simulink model "simple_control"  (R2022b)
settings: Solver=FixedStepDiscrete  StartTime=0.0  StopTime=300  FixedStep=0.01  RelTol=1e-3
model workspace (MAT data in the model file):
  BASE_LENGTH = 0.05
libraries: mobileRoboticsTrainingLib x7
settings Model: NumberOfSteps=10  PacingRate=0.300000  Creator=Amin Fadel  LastModifiedBy=Amin Fadel

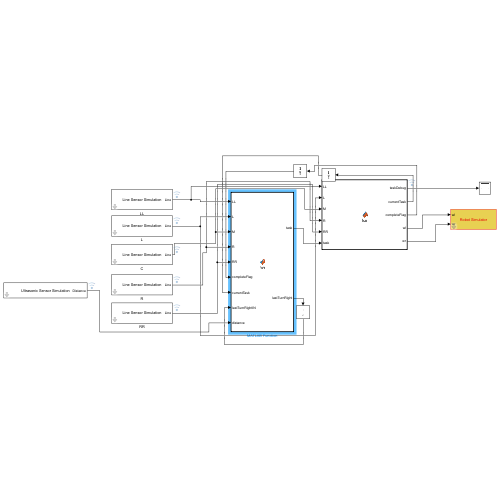
[thumbnail: Simulink's stored preview of the top-level diagram]
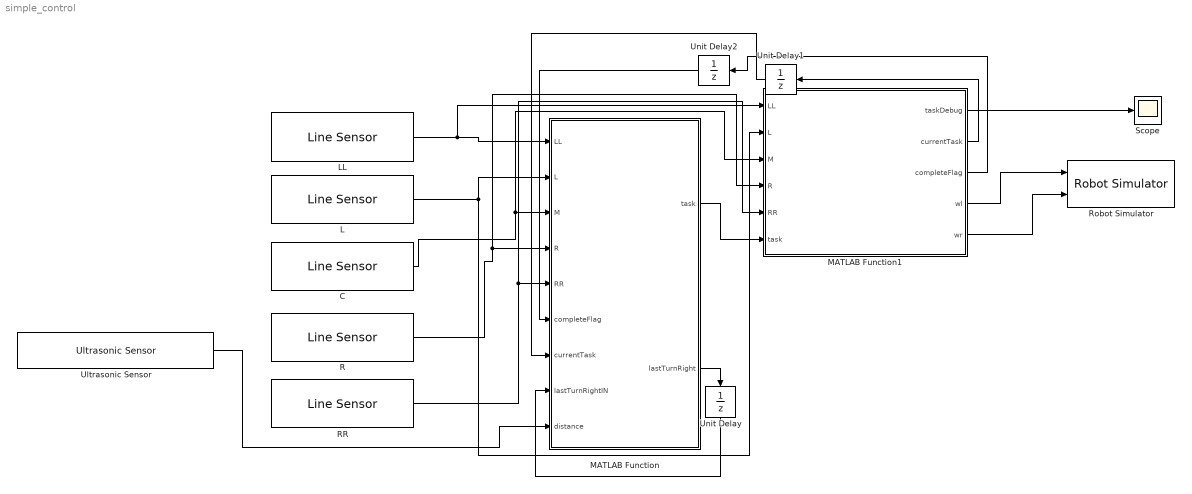
== system simple_control ==
  C : mobileRoboticsTrainingLib/Line Sensor  mapVariable=mapForSim  envVal=0  lineVal=1  sensOff=[BASE_LENGTH+0.05 0]
      settings: SourceProductName=Mobile Robotics Training Library
  L : mobileRoboticsTrainingLib/Line Sensor  mapVariable=mapForSim  envVal=0  lineVal=1  sensOff=[BASE_LENGTH 0.04]
      settings: SourceProductName=Mobile Robotics Training Library
  LL : mobileRoboticsTrainingLib/Line Sensor  mapVariable=mapForSim  envVal=0  lineVal=1  sensOff=[BASE_LENGTH 0.1]
      settings: SourceProductName=Mobile Robotics Training Library
  MATLAB Function : MATLAB Function  TreatAsAtomicUnit=on
  MATLAB Function1 : MATLAB Function  TreatAsAtomicUnit=on
  R : mobileRoboticsTrainingLib/Line Sensor  mapVariable=mapForSim  envVal=0  lineVal=1  sensOff=[BASE_LENGTH -0.04]
      settings: SourceProductName=Mobile Robotics Training Library
  RR : mobileRoboticsTrainingLib/Line Sensor  mapVariable=mapForSim  envVal=0  lineVal=1  sensOff=[BASE_LENGTH -0.1]
      settings: SourceProductName=Mobile Robotics Training Library
  Robot Simulator : mobileRoboticsTrainingLib/Robot Simulator  Priority=99  mapVar=mapForSim  startX=0.10496  startY=1.4665  startTheta=0  axleLength=0.1  wheelR=0.05
  Scope : Scope
  Ultrasonic Sensor : mobileRoboticsTrainingLib/Ultrasonic Sensor  mapVar=mapForSim  maxSenRange=2  minSenRange=0.02  senRes=0.01  sensOff=[BASE_LENGTH+0.06 0]
      settings: SourceProductName=Mobile Robotics Training Library
  Unit Delay : UnitDelay  SampleTime=-1  HasFrameUpgradeWarning=on
  Unit Delay1 : UnitDelay  SampleTime=-1  HasFrameUpgradeWarning=on
  Unit Delay2 : UnitDelay  SampleTime=-1  HasFrameUpgradeWarning=on
  wires:
  LL/1 -> MATLAB Function1/1(LL), MATLAB Function/1(LL)
  L/1 -> MATLAB Function/2(L), MATLAB Function1/2(L)
  C/1 -> MATLAB Function1/3(M), MATLAB Function/3(M)
  R/1 -> MATLAB Function1/4(R), MATLAB Function/4(R)
  RR/1 -> MATLAB Function1/5(RR), MATLAB Function/5(RR)
  MATLAB Function/1(task) -> MATLAB Function1/6(task)
  MATLAB Function/2(lastTurnRight) -> Unit Delay/1
  MATLAB Function1/3(completeFlag) -> Unit Delay2/1
  MATLAB Function1/2(currentTask) -> Unit Delay1/1
  MATLAB Function1/4(wl) -> Robot Simulator/1
  MATLAB Function1/5(wr) -> Robot Simulator/2
  Unit Delay/1 -> MATLAB Function/8(lastTurnRightIN)
  Unit Delay1/1 -> MATLAB Function/7(currentTask)
  Unit Delay2/1 -> MATLAB Function/6(completeFlag)
  MATLAB Function1/1(taskDebug) -> Scope/1
  Ultrasonic Sensor/1 -> MATLAB Function/9(distance)

== matlab function simple_control/MATLAB Function1 ==
  data: taskDebug output; LL input; L input; M input; R input; RR input; task input string; currentTask output string; completeFlag output; wl output; wr output
function [taskDebug, currentTask, completeFlag, wl,wr]= fcn(LL,L,M,R,RR,task)

currentTask = task;
taskDebug = 0;
completeFlag = 1;
wr = 1;
wl = 1;
if(strcmp(task,"turn"))
    taskDebug = 10;
    if(LL == 0 && L == 0 && M == 1 && R == 0 && RR == 0)
        completeFlag = 1;
        return;
    else
        wr = 3;
        wl = -3;
        completeFlag = 0;
    end
end

if(strcmp(task,"forward"))
    taskDebug = 0;
    wr = 3;
    wl = 3;
    completeFlag = 1;
end

if(strcmp(task,"turnSharpLeft"))
    taskDebug = -2;
    if(LL == 0 && M == 1 && RR == 0)
        completeFlag = 1;
        return;
    else
        wr = 3;
        wl = 1;
        completeFlag = 0;
    end
end

if(strcmp(task,"turnSharpRight"))
    taskDebug = 2;
    if(LL == 0 &&  M == 1 && RR == 0)
        completeFlag = 1;
        return;
    else
        wr = 1;
        wl = 3;
        completeFlag = 0;
    end
end

if(strcmp(task,"turnLeft"))
    taskDebug = -1;
    wr = 3;
    wl = 1;
    completeFlag = 1;
end

if(strcmp(task,"turnRight"))
    taskDebug = 1;
    wr = 1;
    wl = 3;
    completeFlag = 1;
end

== matlab function simple_control/MATLAB Function ==
  data: LL input; task output string; L input; M input; R input; RR input; completeFlag input; currentTask input string; lastTurnRight output; lastTurnRightIN input; distance input
function [task,  lastTurnRight]= fcn(LL,L,M,R,RR, completeFlag, currentTask,lastTurnRightIN, distance)

task = "forward";
lastTurnRight = lastTurnRightIN;
if (completeFlag == 0)
    task = currentTask;
else
    if (distance < 0.03 && distance > 0)
        task = "turn";
    elseif (LL == 1 && L == 1  && R == 1 && RR == 1 && lastTurnRightIN == 1)
        lastTurnRight = 0;
        task = "turnSharpLeft";
    elseif (LL == 1 && L == 1 && R == 1 && RR == 1 && lastTurnRightIN == 0)
        lastTurnRight = 1;
        task = "turnSharpRight";
    elseif(RR == 1 && R == 1 && M == 1)
        task = "turnSharpRight";
        lastTurnRight = 1;
    elseif(LL == 1 && L == 1 && M == 1)
        task = "turnSharpLeft";
        lastTurnRight = 0;
    elseif(RR == 1 && R == 1 && M == 0)
        task = "turnSharpRight";
    elseif(LL == 1 && L == 1 && M == 0)
        task = "turnSharpLeft";
    elseif(M == 1)
        task = "forward";
    elseif(L == 1)
        task = "turnLeft";
    elseif(R == 1)
        task = "turnRight";
    end
end
